simulink model "TailSitter_waypoints"  (R2018b)
settings: Solver=VariableStepAuto  StartTime=0.0  StopTime=500  RelTol=1e-3
values from neighbouring files (symbols this model uses):
  p =     [ds.mat]    (also in vxs.mat)
undefined symbols (not defined in the file or in its folder): quatnormalize
libraries: aerolibutil x18, simulink x8, sharedtransform x4, vrlib x3, sharedutil x3, simulink_extras x2, peGeneralControl x1, aerolibanim x1, aerolibanimutils x1
(part 1 of 2)
settings Model: Creator=Robert  LastModifiedBy=Robert

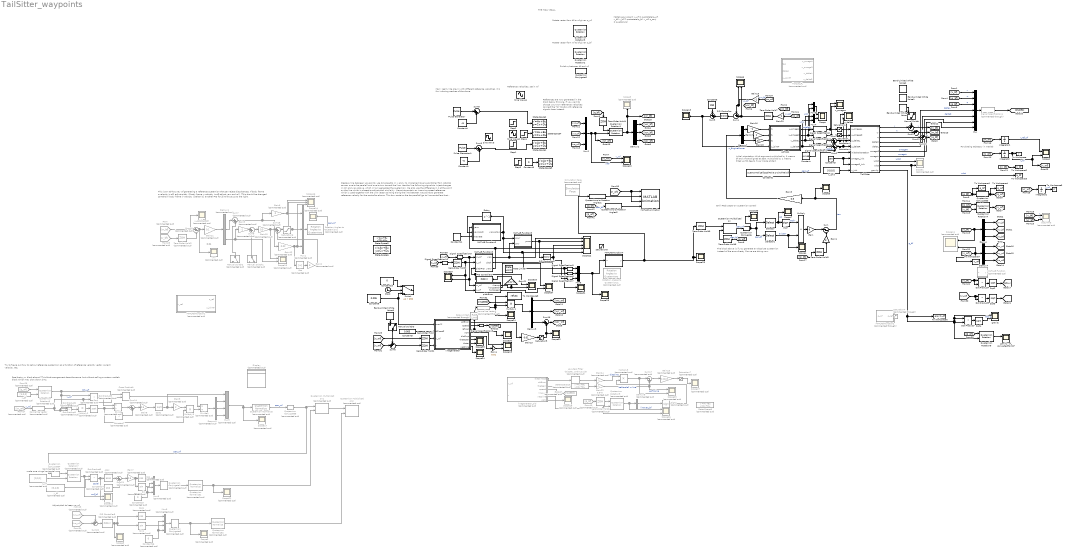
== system TailSitter_waypoints ==
  note: 0.01
  note: The block above is if you generate an absolute
      | quaternion instead of the error directy like we are doing now.
  note: References are now generated in the
      |  block below this one. If you want to
      | choose your own referrence velocities
      | connect the "to" blocks with reference
      | signals here instead.
  note: Create a line between waypoints, use 2d projectio in x and y to implement dual p-controller from robotics course, one to be paralell and one to turn toward the line.
      | Use the line following signals to inject changes in roll and yaw above, which in turn generates the quaternion.
      | We also use the difference in z at the point on the line which is closest to adjust pitch similairly.
      | Wapoints contain an incoming speed reference, which is used together with the unit vector pointing along the line between waypoints to generate reference velocity for the
      | controller above. This box contains the be parallell/go to line controllers that modify
      | the above generated signals.
      | I use low pass filters on the line vector and speed to avoid sharp jumps
      | when switching waypoints.scope
  note: Initial orientation; third argument multiplied
      | by 0 means bf and wf are aligned at start,
      | multiplied by 1 means tilted up 90 deg to
      | hiver mode at start,
  note: Man I really like playin with different reference
      | velocities, it is fun inducing crashes of the drone
  note: This is an ad-hoc way of generating a reference quaternion that can reject disturbances.
      | If body frame z-velocity is off, adjust pitch. If body frame y-velocity is off adjust yaw and roll. (This should be changed somehow)
      | body frame x-velocity is taken by another PID for joint thrust up to the right.
  note: THE HOLY GRAIL
  note: Reference velocities, set in wf
  note: For plotting trajectory in matlab
  note: Emil Fresk paper on quaternion control
  note: Rotate vector from bf to wf given q_wf
  note: Switch q between bf and wf
  note: Rotate vector from wf to bf given q_bf
  note: Matlab equivalent:
      |
      | v_wf = quatrotate(q_wf, v_bf)
      |
      |
      |
      |
      | v_bf = quatrotate(q_bf, v_wf)
      |
      |
      |
      |
      |
      |
      |
      | q_conj = quatconj(q)
  note: Adjust pitch to keep vzr_wf
  note: make sure wings horisontal
  note: See that q_uv block above? This block arangement does the same, but without calling a custom matlab block which may slow down sims.
  note: Try to figure out how to set our reference quaternion as a function of reference velocity vector, current velocity, etc.
  Abs : Abs  Commented=on
  Acos : Trigonometry  Commented=on  Operator=acos
  AdHoc1 : MATLAB Function  TreatAsAtomicUnit=on
  Band-Limited White Noise : simulink/Sources/Band-Limited White Noise  Cov=[0.01]  Ts=0.2  seed=[23343]
  Band-Limited White Noise1 : simulink/Sources/Band-Limited White Noise  Cov=[0.01]  Ts=0.1  seed=[23342]
  Band-Limited White Noise2 : simulink/Sources/Band-Limited White Noise  Cov=[0.01]  Ts=0.1  seed=[23341]
  Band-Limited White Noise3 : simulink/Sources/Band-Limited White Noise  Cov=[0.01 0.01 0.01]  Ts=p.Ts  seed=[23341]
  Clock : Clock
  Constant : Constant  Value=-0.195
  Constant1 : Constant  Value=-5
  Constant10 : Constant  Value=0  SampleTime=p.Ts
  Constant11 : Constant  Value=0.04*10
  Constant14 : Constant  Commented=on  Value=pi/2
  Constant15 : Constant  Commented=on  Value=0
  Constant16 : Constant  Commented=on  Value=0
  Constant2 : Constant  Value=quatnormalize([cosd(45),0,1*sind(45),0])  VectorParams1D=off
  Constant3 : Constant  Value=290
  Constant4 : Constant  Value=-6
  Constant5 : Constant  Value=0.005  SampleTime=p.Ts
  Constant6 : Constant  Value=290
  Constant7 : Constant  Commented=on
  Constant8 : Constant  Value=0.005  SampleTime=p.Ts
  Constant9 : Constant  Value=0
  Cos : Trigonometry  Commented=on  Operator=cos
  Cos1 : Trigonometry  Commented=on  Operator=cos
  Cross Product1 : vrlib/Utilities/Cross Product  Commented=on
      settings: SourceProductBaseCode=VR
  Delay : Delay  DelayLength=1
  Demux{,2..4,7} (5 alike) : Demux  Outputs=3
  Demux1 : Demux  Commented=on  Outputs=3
  Demux5 : Demux  Commented=on  Outputs=3
  Demux8 : Demux  Commented=on  Outputs=3
  Display : Display  Commented=on
  Divide : Product  Commented=on  Inputs=*/
  Divide1 : Product  Commented=on  Inputs=*/
  Dot Product{1..3,6} (4 alike) : DotProduct  Commented=on  InputSameDT=on  OutDataTypeStr=Inherit: Inherit via internal rule
  Dot Product4 : DotProduct  InputSameDT=on  OutDataTypeStr=Inherit: Inherit via internal rule
  Dot Product5 : DotProduct  InputSameDT=on  OutDataTypeStr=Inherit: Inherit via internal rule
  Dot Product7 : DotProduct  InputSameDT=on  OutDataTypeStr=Inherit: Inherit via internal rule
  From : From  Commented=on  GotoTag=vr_bf
  From26 : From  Commented=on  GotoTag=q_wf
  From27 : From  Commented=on  GotoTag=vr_wf
  From28 : From  Commented=on  GotoTag=v_bf
  From33 : From  Commented=on  GotoTag=vz_wf
  From34 : From  Commented=on  GotoTag=vzr_wf
  From40 : From  Commented=on  GotoTag=q_bf
  Gain : Gain  Gain=8
  Gain1 : Gain  Gain=3
  Gain11 : Gain  Commented=on  Gain=0.1
  Gain12 : Gain  Commented=on  Gain=0.02
  Gain13 : Gain  Gain=0.01
  Gain15 : Gain  Commented=on  Gain=0.5
  Gain16 : Gain  Gain=-1
  Gain17 : Gain
  Gain18 : Gain  Gain=-30
  Gain19 : Gain  Gain=-1
  Gain2 : Gain  Commented=on  Gain=5
  Gain20 : Gain  Gain=-1
  Gain21 : Gain  Gain=-0.01*0
  Gain22 : Gain  Commented=on  Gain=0.5*0
  Gain23 : Gain  Commented=on  Gain=0.0025
  Gain24 : Gain  Commented=on  Gain=-1
  Gain3 : Gain  Gain=0.5
  Gain4 : Gain  Gain=0.01
  Gain5 : Gain  Commented=on  Gain=-1
  Gain6 : Gain  Commented=on  Gain=0
  Gain7 : Gain  Commented=on  Gain=0.5
  Gain8 : Gain  Commented=on  Gain=0.5
  Gain9 : Gain  Commented=on  Gain=2
  Goto27 : Goto  Commented=on  GotoTag=rspeed
  Integrator : Integrator
  Integrator1 : Integrator
  Integrator2 : Integrator
  Low-Pass Filter (Discrete or Continuous)3 : peGeneralControl/Low-Pass Filter (Discrete or Continuous)  Commented=on  K=1  T=2  B=inf  A=-inf  Ts=-1
  MATLAB Animation : aerolibanim/MATLAB Animation  Tag=Matlab Animation 6 DOF  Vehicles=2  Geometries={'astredwedge.mat',a}  BoundingBoxCoordinates=[-50,50,-50,50,-50,50]  CameraOffset=[-150,0,-50]  CameraViewAngle=3  SampleTime=0.2  FigurePosition=[7,613,791,375]
      settings: SourceProductName=Aerospace Blockset  SourceProductBaseCode=AE
  MATLAB Function : MATLAB Function  Commented=on  TreatAsAtomicUnit=on
  MATLAB Function1 : MATLAB Function  Commented=on  TreatAsAtomicUnit=on
  MATLAB Function2 : MATLAB Function  Commented=through  TreatAsAtomicUnit=on
  MATLAB Function3 : MATLAB Function  TreatAsAtomicUnit=on
  MATLAB Function4 : MATLAB Function  TreatAsAtomicUnit=on
  MATLAB Function5 : MATLAB Function  TreatAsAtomicUnit=on
  MATLAB Function6 : MATLAB Function  TreatAsAtomicUnit=on
  Manual Switch : ManualSwitch  CurrentSetting=0
  Manual Switch1 : ManualSwitch  Commented=on  CurrentSetting=0
  Manual Switch2 : ManualSwitch  Commented=on  CurrentSetting=0
  Manual Switch3 : ManualSwitch  CurrentSetting=0
  Multiply : Product
  Multiply1 : Product
  Multiply2 : Product  Commented=on
  Multiply3 : Product  Commented=on
  Multiply5 : Product  Commented=on
  Mux : Mux  Inputs=7
  Mux1 : Mux  Commented=on  Inputs=3
  Mux2 : Mux  Inputs=3
  Mux3 : Mux  Inputs=2
  Mux4 : Mux  Inputs=2
  Mux5 : Mux  Commented=on
  Mux6 : Mux  Inputs=3
  Mux8 : Mux  Commented=on
  Mux9 : Mux  Commented=on
  Normalize Vector : vrlib/Utilities/Normalize Vector  Commented=on  maxzero=0
      settings: SourceProductName=Simulink 3D Animation  SourceProductBaseCode=VR
  Normalize Vector1 : vrlib/Utilities/Normalize Vector  Commented=through  maxzero=0
      settings: SourceProductName=Simulink 3D Animation  SourceProductBaseCode=VR
  PID Controller : simulink/Continuous/PID Controller  Controller=PID  Form=Parallel  TimeDomain=Discrete-time  SampleTime=-1  IntegratorMethod=Forward Euler  FilterMethod=Forward Euler  ControllerParametersSource=internal  P=150*2  I=50*0.5  D=50  UseFilter=off  N=100  TunerSelectOption=Transfer Function Based (PID Tuner App)  InitialConditionSource=internal  InitialConditionForIntegrator=0  InitialConditionForFilter=0  DifferentiatorICPrevScaledInput=0  ExternalReset=none  TrackingMode=off  Kt=1  LimitOutput=on  UpperSaturationLimit=4000-290  LowerSaturationLimit=-290  LinearizeAsGain=on  AntiWindupMode=clamping  Kb=1  POutMin=[]  POutMax=[]  IOutMin=[]  IOutMax=[]  DOutMin=[]  DOutMax=[]  NOutMin=[]  NOutMax=[]  SumOutMin=[]  SumOutMax=[]  SaturationOutMin=[]  SaturationOutMax=[]  PParamMin=[]  PParamMax=[]  IParamMin=[]  IParamMax=[]  DParamMin=[]  DParamMax=[]  NParamMin=[]  NParamMax=[]  KbParamMin=[]  KbParamMax=[]  KtParamMin=[]  KtParamMax=[]  KbOutMin=[]  KbOutMax=[]  KtOutMin=[]  KtOutMax=[]  IntegratorOutMin=[]  IntegratorOutMax=[]  FilterOutMin=[]  FilterOutMax=[]  SumI1OutMin=[]  SumI1OutMax=[]  SumI2OutMin=[]  SumI2OutMax=[]  SumI3OutMin=[]  SumI3OutMax=[]  SumI4OutMin=[]  SumI4OutMax=[]  SumDOutMin=[]  SumDOutMax=[]  DifferentiatorOutMin=[]  DifferentiatorOutMax=[]  FilterDiffOutCoefMin=[]  FilterDiffOutCoefMax=[]  ReciprocalOutMin=[]  ReciprocalOutMax=[]  SumDenOutMin=[]  SumDenOutMax=[]  SumNumOutMin=[]  SumNumOutMax=[]  DivideOutMin=[]  DivideOutMax=[]  IntegratorContinuousStateAttributes=''  IntegratorStateMustResolveToSignalObject=off  IntegratorRTWStateStorageClass=Auto  FilterContinuousStateAttributes=''  FilterStateMustResolveToSignalObject=off  FilterRTWStateStorageClass=Auto  ParallelPVariant=InternalParameters  IdealPVariant=Disabled  IVariant=InternalParameters  DVariant=InternalParameters  IntegratorVariant=Discrete  SatVariant=Enabled  AWVariant=DiscClampingParallel  PCopyVariant=Disabled  TRVariant=Disabled  FdbkBlocksVariant=Forward  IdealPFdbkVariant=Disabled  SatFdbkVariant=Disabled  DerivativeFilterVariant=Differentiator  NVariant=Passthrough  NCopyVariant=Disabled_SignalSpec  FilterICVariant=InternalICsDifferentiator  IntegratorICVariant=InternalICs  ExternalResetVariant=Disabled  TRSumVariant=Passthrough  SumFdbkVariant=Disabled  SumVariant=Sum_PID
  PID Controller1 : simulink/Continuous/PID Controller  Controller=PID  Form=Parallel  TimeDomain=Discrete-time  SampleTime=-1  IntegratorMethod=Forward Euler  FilterMethod=Forward Euler  ControllerParametersSource=internal  P=2*1.25*0  I=0.1*2  D=1*0  UseFilter=off  N=100  TunerSelectOption=Transfer Function Based (PID Tuner App)  InitialConditionSource=internal  InitialConditionForIntegrator=0  InitialConditionForFilter=0  DifferentiatorICPrevScaledInput=0  ExternalReset=none  TrackingMode=off  Kt=1  LimitOutput=on  UpperSaturationLimit=deg2rad(9)  LowerSaturationLimit=-deg2rad(9)  LinearizeAsGain=on  AntiWindupMode=clamping  Kb=1  POutMin=[]  POutMax=[]  IOutMin=[]  IOutMax=[]  DOutMin=[]  DOutMax=[]  NOutMin=[]  NOutMax=[]  SumOutMin=[]  SumOutMax=[]  SaturationOutMin=[]  SaturationOutMax=[]  PParamMin=[]  PParamMax=[]  IParamMin=[]  IParamMax=[]  DParamMin=[]  DParamMax=[]  NParamMin=[]  NParamMax=[]  KbParamMin=[]  KbParamMax=[]  KtParamMin=[]  KtParamMax=[]  KbOutMin=[]  KbOutMax=[]  KtOutMin=[]  KtOutMax=[]  IntegratorOutMin=[]  IntegratorOutMax=[]  FilterOutMin=[]  FilterOutMax=[]  SumI1OutMin=[]  SumI1OutMax=[]  SumI2OutMin=[]  SumI2OutMax=[]  SumI3OutMin=[]  SumI3OutMax=[]  SumI4OutMin=[]  SumI4OutMax=[]  SumDOutMin=[]  SumDOutMax=[]  DifferentiatorOutMin=[]  DifferentiatorOutMax=[]  FilterDiffOutCoefMin=[]  FilterDiffOutCoefMax=[]  ReciprocalOutMin=[]  ReciprocalOutMax=[]  SumDenOutMin=[]  SumDenOutMax=[]  SumNumOutMin=[]  SumNumOutMax=[]  DivideOutMin=[]  DivideOutMax=[]  IntegratorContinuousStateAttributes=''  IntegratorStateMustResolveToSignalObject=off  IntegratorRTWStateStorageClass=Auto  FilterContinuousStateAttributes=''  FilterStateMustResolveToSignalObject=off  FilterRTWStateStorageClass=Auto  ParallelPVariant=InternalParameters  IdealPVariant=Disabled  IVariant=InternalParameters  DVariant=InternalParameters  IntegratorVariant=Discrete  SatVariant=Enabled  AWVariant=DiscClampingParallel  PCopyVariant=Disabled  TRVariant=Disabled  FdbkBlocksVariant=Forward  IdealPFdbkVariant=Disabled  SatFdbkVariant=Disabled  DerivativeFilterVariant=Differentiator  NVariant=Passthrough  NCopyVariant=Disabled_SignalSpec  FilterICVariant=InternalICsDifferentiator  IntegratorICVariant=InternalICs  ExternalResetVariant=Disabled  TRSumVariant=Passthrough  SumFdbkVariant=Disabled  SumVariant=Sum_PID
  PID Controller2 : simulink/Continuous/PID Controller  Controller=PID  Form=Parallel  TimeDomain=Discrete-time  SampleTime=-1  IntegratorMethod=Forward Euler  FilterMethod=Forward Euler  ControllerParametersSource=internal  P=1*0  I=0  D=0.5*0  UseFilter=off  N=100  TunerSelectOption=Transfer Function Based (PID Tuner App)  InitialConditionSource=internal  InitialConditionForIntegrator=0  InitialConditionForFilter=0  DifferentiatorICPrevScaledInput=0  ExternalReset=none  TrackingMode=off  Kt=1  LimitOutput=on  UpperSaturationLimit=deg2rad(50)  LowerSaturationLimit=-deg2rad(50)  LinearizeAsGain=on  AntiWindupMode=clamping  Kb=1  POutMin=[]  POutMax=[]  IOutMin=[]  IOutMax=[]  DOutMin=[]  DOutMax=[]  NOutMin=[]  NOutMax=[]  SumOutMin=[]  SumOutMax=[]  SaturationOutMin=[]  SaturationOutMax=[]  PParamMin=[]  PParamMax=[]  IParamMin=[]  IParamMax=[]  DParamMin=[]  DParamMax=[]  NParamMin=[]  NParamMax=[]  KbParamMin=[]  KbParamMax=[]  KtParamMin=[]  KtParamMax=[]  KbOutMin=[]  KbOutMax=[]  KtOutMin=[]  KtOutMax=[]  IntegratorOutMin=[]  IntegratorOutMax=[]  FilterOutMin=[]  FilterOutMax=[]  SumI1OutMin=[]  SumI1OutMax=[]  SumI2OutMin=[]  SumI2OutMax=[]  SumI3OutMin=[]  SumI3OutMax=[]  SumI4OutMin=[]  SumI4OutMax=[]  SumDOutMin=[]  SumDOutMax=[]  DifferentiatorOutMin=[]  DifferentiatorOutMax=[]  FilterDiffOutCoefMin=[]  FilterDiffOutCoefMax=[]  ReciprocalOutMin=[]  ReciprocalOutMax=[]  SumDenOutMin=[]  SumDenOutMax=[]  SumNumOutMin=[]  SumNumOutMax=[]  DivideOutMin=[]  DivideOutMax=[]  IntegratorContinuousStateAttributes=''  IntegratorStateMustResolveToSignalObject=off  IntegratorRTWStateStorageClass=Auto  FilterContinuousStateAttributes=''  FilterStateMustResolveToSignalObject=off  FilterRTWStateStorageClass=Auto  ParallelPVariant=InternalParameters  IdealPVariant=Disabled  IVariant=InternalParameters  DVariant=InternalParameters  IntegratorVariant=Discrete  SatVariant=Enabled  AWVariant=DiscClampingParallel  PCopyVariant=Disabled  TRVariant=Disabled  FdbkBlocksVariant=Forward  IdealPFdbkVariant=Disabled  SatFdbkVariant=Disabled  DerivativeFilterVariant=Differentiator  NVariant=Passthrough  NCopyVariant=Disabled_SignalSpec  FilterICVariant=InternalICsDifferentiator  IntegratorICVariant=InternalICs  ExternalResetVariant=Disabled  TRSumVariant=Passthrough  SumFdbkVariant=Disabled  SumVariant=Sum_PID
  PID Controller5 : simulink/Continuous/PID Controller  Commented=on  Controller=PID  Form=Parallel  TimeDomain=Continuous-time  SampleTime=-1  IntegratorMethod=Forward Euler  FilterMethod=Forward Euler  ControllerParametersSource=internal  P=0.04*2  I=0  D=0  UseFilter=on  N=100  TunerSelectOption=Transfer Function Based (PID Tuner App)  InitialConditionSource=internal  InitialConditionForIntegrator=0  InitialConditionForFilter=0  DifferentiatorICPrevScaledInput=0  ExternalReset=none  TrackingMode=off  Kt=1  LimitOutput=off  UpperSaturationLimit=inf  LowerSaturationLimit=-inf  LinearizeAsGain=on  AntiWindupMode=none  Kb=1  POutMin=[]  POutMax=[]  IOutMin=[]  IOutMax=[]  DOutMin=[]  DOutMax=[]  NOutMin=[]  NOutMax=[]  SumOutMin=[]  SumOutMax=[]  SaturationOutMin=[]  SaturationOutMax=[]  PParamMin=[]  PParamMax=[]  IParamMin=[]  IParamMax=[]  DParamMin=[]  DParamMax=[]  NParamMin=[]  NParamMax=[]  KbParamMin=[]  KbParamMax=[]  KtParamMin=[]  KtParamMax=[]  KbOutMin=[]  KbOutMax=[]  KtOutMin=[]  KtOutMax=[]  IntegratorOutMin=[]  IntegratorOutMax=[]  FilterOutMin=[]  FilterOutMax=[]  SumI1OutMin=[]  SumI1OutMax=[]  SumI2OutMin=[]  SumI2OutMax=[]  SumI3OutMin=[]  SumI3OutMax=[]  SumI4OutMin=[]  SumI4OutMax=[]  SumDOutMin=[]  SumDOutMax=[]  DifferentiatorOutMin=[]  DifferentiatorOutMax=[]  FilterDiffOutCoefMin=[]  FilterDiffOutCoefMax=[]  ReciprocalOutMin=[]  ReciprocalOutMax=[]  SumDenOutMin=[]  SumDenOutMax=[]  SumNumOutMin=[]  SumNumOutMax=[]  DivideOutMin=[]  DivideOutMax=[]  IntegratorContinuousStateAttributes=''  IntegratorStateMustResolveToSignalObject=off  IntegratorRTWStateStorageClass=Auto  FilterContinuousStateAttributes=''  FilterStateMustResolveToSignalObject=off  FilterRTWStateStorageClass=Auto  ParallelPVariant=InternalParameters  IdealPVariant=Disabled  IVariant=InternalParameters  DVariant=InternalParameters  IntegratorVariant=Continuous  SatVariant=Disabled  AWVariant=Passthrough  PCopyVariant=Disabled  TRVariant=Disabled  FdbkBlocksVariant=Forward  IdealPFdbkVariant=Disabled  SatFdbkVariant=Disabled  DerivativeFilterVariant=ContFilter  NVariant=InternalParameters  NCopyVariant=Disabled  FilterICVariant=InternalICsFilter  IntegratorICVariant=InternalICs  ExternalResetVariant=Disabled  TRSumVariant=Passthrough  SumFdbkVariant=Disabled  SumVariant=Sum_PID
  Pulse Generator : DiscretePulseGenerator  PulseType=Time based  Amplitude=12  Period=50  PulseWidth=50
  Pulse Generator1 : DiscretePulseGenerator  PulseType=Time based  Amplitude=8  Period=60  PulseWidth=50  PhaseDelay=30
  Quaternion Conjugate : aerolibutil/Quaternion Conjugate
      settings: SourceProductName=Aerospace Blockset  SourceProductBaseCode=AE
  Quaternion Conjugate{1,4..6} (4 alike) : aerolibutil/Quaternion Conjugate  Commented=on
      settings: SourceProductName=Aerospace Blockset  SourceProductBaseCode=AE
  Quaternion Conjugate2 : aerolibutil/Quaternion Conjugate
      settings: SourceProductName=Aerospace Blockset  SourceProductBaseCode=AE
  Quaternion Conjugate3 : aerolibutil/Quaternion Conjugate
      settings: SourceProductName=Aerospace Blockset  SourceProductBaseCode=AE
  Quaternion Multiplication : aerolibutil/Quaternion Multiplication
  Quaternion Multiplication1 : aerolibutil/Quaternion Multiplication  Commented=on
  Quaternion Multiplication2 : aerolibutil/Quaternion Multiplication  Commented=on
  Quaternion Normalize : sharedutil/Quaternion Normalize  Commented=on  aMode=aMode
      settings: SourceProductName=Aerospace Blockset  SourceProductBaseCode=AE
  Quaternion Normalize1 : sharedutil/Quaternion Normalize  Commented=on  aMode=aMode
      settings: SourceProductName=Aerospace Blockset  SourceProductBaseCode=AE
  Quaternion Normalize2 : sharedutil/Quaternion Normalize  Commented=on  aMode=aMode
      settings: SourceProductName=Aerospace Blockset  SourceProductBaseCode=AE
  Quaternion Rotation{1..4,8} (5 alike) : aerolibutil/Quaternion Rotation
  Quaternion Rotation5 : aerolibutil/Quaternion Rotation  Commented=on
  Quaternion Rotation7 : aerolibutil/Quaternion Rotation  Commented=on
  Quaternion Rotation9 : aerolibutil/Quaternion Rotation  Commented=on
  Quaternions to Rotation Angles1 : sharedtransform/Quaternions to Rotation Angles  rotationOrder=XYZ  aMode=aMode
      settings: SourceProductBaseCode=AE
  Quaternions to Rotation Angles2 : sharedtransform/Quaternions to Rotation Angles  rotationOrder=XYZ  aMode=aMode
      settings: SourceProductBaseCode=AE
  Rate Limiter : RateLimiter  RisingSlewLimit=0.1  FallingSlewLimit=-0.1  SampleTimeMode=inherited
  Rate Limiter1 : RateLimiter  Commented=through  RisingSlewLimit=0.03  FallingSlewLimit=-0.03  SampleTimeMode=inherited
  Rotation Angles to Quaternions : sharedtransform/Rotation Angles to Quaternions  Commented=on  rotationOrder=ZYX  aMode=aMode
      settings: SourceProductName=Aerospace Blockset  SourceProductBaseCode=AE
  Rotation Angles to Quaternions1 : sharedtransform/Rotation Angles to Quaternions  Commented=on  rotationOrder=ZYX  aMode=aMode
      settings: SourceProductName=Aerospace Blockset  SourceProductBaseCode=AE
  Saturation : Saturate  UpperLimit=1000  LowerLimit=0
  Saturation1 : Saturate  UpperLimit=1000  LowerLimit=0
  Saturation2 : Saturate  UpperLimit=1  LowerLimit=-1
  Saturation3 : Saturate  UpperLimit=1  LowerLimit=-1
  Saturation4 : Saturate  Commented=through
  Saturation5 : Saturate  UpperLimit=0.01  LowerLimit=-0.01
  Saturation6 : Saturate  Commented=on  UpperLimit=1  LowerLimit=-1
  Saturation7 : Saturate  Commented=on
  Saturation8 : Saturate  UpperLimit=deg2rad(50)  LowerLimit=-deg2rad(50)
  Scope{,2,6,10,19..20,29,33,37} (9 alike) : Scope  NumInputPorts=2
  Scope{1,11..12,15,23,26} (6 alike) : Scope  Commented=on  NumInputPorts=2
  Scope{4..5,7,13,24..25,28,30..32,34..35} (12 alike) : Scope
  Scope{3,8..9,14,17..18,21,27} (8 alike) : Scope  Commented=on
  Scope16 : Scope  Commented=on  NumInputPorts=3
  Scope22 : Scope  NumInputPorts=5
  Selector : Selector  IndexMode=Zero-based  InputPortWidth=4  IndexOptions=Index vector (dialog)  Indices=[0 ]  OutputSizes=1
  Selector1 : Selector  IndexMode=Zero-based  InputPortWidth=4  IndexOptions=Index vector (dialog)  Indices=[1:3]  OutputSizes=1
  Sign : Signum
  Sign2 : Signum  Commented=on
  Signal Specification{,1..3,5..8} (8 alike) : SignalSpecification  Dimensions=1
  Signal Specification10 : SignalSpecification  Dimensions=3
  Signal Specification4 : SignalSpecification  Commented=through  Dimensions=14
  Signal Specification9 : SignalSpecification  Dimensions=3
  Simulation Pace : aerolibanimutils/Simulation Pace  Commented=on  SimulationPace=2  SleepMode=Auto  OutputPaceError=off  SampleTime=1/30
  Sin : Trigonometry  Commented=on
  Sin1 : Trigonometry  Commented=on
  Sine Wave : Sin  Amplitude=-2  Frequency=1/15  Phase=pi/2  SampleTime=0
  Sine Wave1 : Sin  Amplitude=-8  Frequency=1/20  SampleTime=0
  Sine Wave2 : Sin  Amplitude=10  Frequency=1/45  SampleTime=0
  Sqrt : Sqrt  Commented=on  SaturateOnIntegerOverflow=on
  Sqrt1 : Sqrt  Commented=on  SaturateOnIntegerOverflow=on
  Sqrt2 : Sqrt  SaturateOnIntegerOverflow=on
  Sqrt3 : Sqrt  SaturateOnIntegerOverflow=on
  Sqrt4 : Sqrt  SaturateOnIntegerOverflow=on
  State-Space1 : StateSpace  A=-1/5  B=1/5  D=0  InitialCondition=0
  State-Space10 : StateSpace  Commented=on  A=-1/15  B=1/15  D=0  InitialCondition=0
  State-Space2 : StateSpace  A=-1/15  B=1/15  D=0  InitialCondition=0
  State-Space3 : StateSpace  A=-1/15  B=1/15  D=0  InitialCondition=0
  State-Space4 : StateSpace  A=-1/15  B=1/15  D=0  InitialCondition=0
  State-Space5 : StateSpace  A=-1/5  B=1/5  D=0  InitialCondition=0
  State-Space6 : StateSpace  A=-1/2*eye(3)  B=1/2*eye(3)  C=eye(3)  D=0*eye(3)  InitialCondition=0
  State-Space9 : StateSpace  Commented=on  A=-1/4  B=1/4  D=0  InitialCondition=0
  Step1 : Step  Time=20  After=-10  SampleTime=0
  Step2 : Step  Time=100  After=5  SampleTime=0
  Step3 : Step  Time=30  Before=-1  After=0  SampleTime=0
  Step4 : Step  Time=60  After=18  SampleTime=0
  Sum : Sum  Inputs=|--
  Sum{1..3,8,16} (5 alike) : Sum  Inputs=|++
  Sum10 : Sum  Commented=on  Inputs=|+-
  Sum{5..6,11..13} (5 alike) : Sum  Inputs=++|
  Sum{7,9,14..15} (4 alike) : Sum  Commented=on  Inputs=|++
  Sum17 : Sum  Commented=on  Inputs=|-+
  Sum21 : Sum  Commented=on  Inputs=|+-
  Sum22 : Sum  Commented=on  Inputs=-+|
  Sum4 : Sum  Inputs=+-|
  Switch : Switch  Criteria=u2 > Threshold  Threshold=250
  TailSitter : Subsystem
  To Workspace : ToWorkspace  VariableName=r  SaveFormat=Timeseries  SampleTime=p.Ts_log
  To Workspace1 : ToWorkspace  VariableName=q_bf  SaveFormat=Timeseries  SampleTime=p.Ts_log
  To Workspace2 : ToWorkspace  VariableName=v_bf  SaveFormat=Timeseries  SampleTime=p.Ts_log
  To Workspace3 : ToWorkspace  VariableName=a_bf  SaveFormat=Timeseries  SampleTime=p.Ts_log
  To Workspace4 : ToWorkspace  VariableName=q_wf  SaveFormat=Timeseries  SampleTime=p.Ts_log
  To Workspace5 : ToWorkspace  VariableName=rr  SaveFormat=Timeseries  SampleTime=p.Ts_log
  To Workspace6 : ToWorkspace  VariableName=gravity_bf  SaveFormat=Timeseries  SampleTime=p.Ts_log
  To Workspace7 : ToWorkspace  VariableName=v_wf  SaveFormat=Timeseries  SampleTime=p.Ts_log
  To Workspace8 : ToWorkspace  VariableName=refvec  SaveFormat=Timeseries  SampleTime=p.Ts_log
  Torque_FL : MATLAB Function  Commented=on  TreatAsAtomicUnit=on
  Zero-Order Hold{,1,3..5,7..9} (8 alike) : ZeroOrderHold  SampleTime=p.Ts
  Zero-Order Hold2 : ZeroOrderHold  Commented=on  SampleTime=p.Ts
  Zero-Order Hold6 : ZeroOrderHold  Commented=on  SampleTime=p.Ts
  bodyfrme : Scope  Commented=on  NumInputPorts=2
  gravity : Scope  NumInputPorts=2
  gravity_wf_convertedfrombf : Scope  NumInputPorts=2
  linegenerator : MATLAB Function  TreatAsAtomicUnit=on
  linegenerator_old : MATLAB Function  Commented=on  TreatAsAtomicUnit=on
  pitchError : MATLAB Function  TreatAsAtomicUnit=on
  u_deltas : Scope  NumInputPorts=2
  u_omegas : Scope  NumInputPorts=2
  v_isnit : Constant  Value=[0,0,0]
  "v_ref_bf_attctrl " : Scope  Commented=on
  vr-v : Scope  Commented=on
  x_bf : Constant  Commented=on  Value=[1,0,0]
  y_bf : Constant  Commented=on  Value=[0,1,0]
  z_wf : Constant  Commented=on  Value=[0,0,1]
  wires:
  Selector1/1 -> Scope4/1, Multiply/2  "axiserr"
  Selector/1 -> Scope7/1, Sign/1  "q0"
  Sign/1 -> Multiply/1  "rotdir"
  Gain1/1 -> Sum/2
  Sum5/1 -> AdHoc1/4(u_jointT), Scope13/1  "u_EnginePower"
  Constant3/1 -> TailSitter/7(omegaR_init), TailSitter/6(omegaL_init)
  Sum11/1 -> [v_bf]  "v"
  TailSitter/8(wdot) -> Scope1/1  "wdot"
  TailSitter/9(vdot) -> To Workspace3/1, Scope1/2  "vdot"
  Integrator/1 -> [r_wf], Scope2/2, To Workspace/1  "r_wf"
  [v_wf] -> Integrator/1
  v_isnit/1 -> TailSitter/8(v_init)
  Sum4/1 -> PID Controller/1
  Sum/1 -> Scope5/1, Gain3/1  "tao"
  PID Controller/1 -> Sum5/2
  Constant6/1 -> Sum5/1
  Multiply/1 -> Gain/1
  [vzr_wf] -> Gain19/1  "vxr_bf"
  Saturation/1 -> TailSitter/2(u_omegaR)
  Saturation1/1 -> TailSitter/1(u_omegaL)
  TailSitter/3(q) -> Sum13/2
  Mux2/1 -> Scope10/2, [vr_wf], Quaternion Rotation1/2  "vref"
  Quaternion Rotation1/1 -> Demux2/1, [vr_bf], Scope9/1
  Demux2/3 -> [vzr_bf]
  Demux2/2 -> [vyr_bf]
  Demux2/1 -> [vxr_bf]
  Zero-Order Hold7/1 -> Scope6/2, Sum4/2  "vx_bf"
  [v_wf] -> Scope10/1  "v_wf"
  [q_bf] -> Zero-Order Hold4/1
  [q_bf] -> To Workspace1/1, Quaternion Conjugate3/1
  Quaternion Conjugate3/1 -> To Workspace4/1, [q_wf]
  [vxr_wf] -> Mux2/1
  [vyr_wf] -> Mux2/2
  [vzr_wf] -> Mux2/3
  [q_wf] -> Quaternion Rotation4/1
  Quaternion Rotation4/1 -> [v_wf]
  [v_bf] -> Quaternion Rotation4/2
  TailSitter/2(w) -> Sum12/2  "w"
  Demux/1 -> [vx_bf]
  Demux/3 -> [vz_bf]
  Demux/2 -> [vy_bf]
  [v_bf] -> Scope11/1, Demux/1
  Demux4/2 -> [vy_wf]
  Demux4/3 -> [vz_wf]
  Demux4/1 -> [vx_wf]
  [v_wf] -> To Workspace7/1, Scope11/2, Demux4/1
  [v_bf] -> To Workspace2/1
  [v_bf] -> Dot Product4/2, Dot Product4/1
  Sqrt2/1 -> [abs_v]
  [vr_wf] -> Integrator1/1
  Integrator1/1 -> Scope2/1  "r_ref_wf"
  [w_bf] -> Zero-Order Hold5/1
  [v_bf] -> bodyfrme/1  "v"
  [vr_bf] -> bodyfrme/2  "vr"
  [vr_wf] -> Integrator2/1
  Integrator2/1 -> To Workspace5/1  "r_wf"
  Dot Product4/1 -> Sqrt2/1
  Gain/1 -> Sum/1
  Constant2/1 -> TailSitter/5(initialOrientation)  "qerr_wf"
  [v_bf] -> Mux/1  "v"
  [w_bf] -> Mux/2  "w"
  [q_bf] -> Mux/3  "q"
  TailSitter/5(deltaL) -> Mux/4  "deltaL"
  TailSitter/4(deltaR) -> Mux/5  "deltaR"
  TailSitter/7(omegaL) -> Mux/6  "omegaL"
  TailSitter/6(omegaR) -> Mux/7  "omegaR"
  AdHoc1/1(u_omegaL) -> Mux3/2, Signal Specification/1  "uWL"
  AdHoc1/2(u_omegaR) -> Mux3/1, Signal Specification1/1
  AdHoc1/3(u_deltaL) -> Mux4/1, Signal Specification2/1  "uWL"
  AdHoc1/4(u_deltaR) -> Signal Specification3/1, Mux4/2  "udeltaL"
  Signal Specification/1 -> u_omegas/1, Saturation1/1
  Signal Specification1/1 -> u_omegas/2, Saturation/1
  Signal Specification2/1 -> Sum1/1
  Signal Specification3/1 -> Sum2/1
  Mux/1 -> Signal Specification4/1
  Sum1/1 -> Saturation2/1
  Signal Specification4/1 -> [states]
  Acos/1 -> Sum21/1
  y_bf/1 -> Dot Product6/2
  Multiply3/1 -> Divide1/2
  Sum22/1 -> PID Controller5/1
  Dot Product3/1 -> Divide/1
  Demux5/2 -> Mux5/3
  Quaternion Conjugate6/1 -> Scope3/1, Quaternion Normalize2/1
  Mux5/1 -> Scope17/1, Quaternion Normalize/1
  From33/1 -> Sum22/1
  Constant15/1 -> Mux8/3, Mux8/4
  Mux8/1 -> Quaternion Conjugate1/1
  Demux5/1 -> Mux5/2
  PID Controller5/1 -> Scope8/1, Cos1/1, Sin1/1
  From27/1 -> Normalize Vector/1  "v_wf"
  Cos1/1 -> Mux9/1
  Quaternion Rotation7/1 -> Scope12/1, Dot Product6/1  "zwf_bf"
  Constant16/1 -> Mux9/2, Mux9/4
  Quaternion Normalize1/1 -> Scope21/1, Quaternion Multiplication1/2
  Gain7/1 -> Sin/1, Cos/1
  Sum21/1 -> Gain7/1
  From34/1 -> Sum22/2
  Mux9/1 -> Quaternion Conjugate6/1
  Cos/1 -> Mux8/1
  Constant14/1 -> Sum21/2
  Sin/1 -> Mux8/2
  Quaternion Normalize2/1 -> Quaternion Multiplication2/2
  Multiply2/1 -> Sqrt/1
  Divide/1 -> Sum14/1
  Quaternion Conjugate1/1 -> Quaternion Normalize1/1
  Sin1/1 -> Mux9/3
  Sqrt1/1 -> Mux5/1, Gain9/1
  Quaternion Conjugate4/1 -> Quaternion Rotation7/1
  Normalize Vector/1 -> Cross Product1/2, Dot Product3/2, Dot Product2/1, Dot Product2/2  "v_wf"
  Quaternion Normalize/1 -> Quaternion Conjugate5/1  "qerr_wf"
  Gain8/1 -> Sqrt1/1
  Cross Product1/1 -> Divide1/1
  Divide1/1 -> Demux5/1
  From26/1 -> Quaternion Rotation5/1
  Sum14/1 -> Gain8/1
  z_wf/1 -> Quaternion Rotation7/2
  Dot Product6/1 -> Scope12/2, Acos/1  "cos(a)"
  Gain9/1 -> Multiply3/1
  Dot Product1/1 -> Multiply2/1
  Constant7/1 -> Sum14/2
  Dot Product2/1 -> Multiply2/2
  Sqrt/1 -> Multiply3/2, Divide/2
  Quaternion Rotation5/1 -> Dot Product3/1, Dot Product1/2, Dot Product1/1, Cross Product1/1  "bfx_wf"
  Demux5/3 -> Mux5/4
  x_bf/1 -> Quaternion Rotation5/2
  Quaternion Multiplication1/1 -> Quaternion Multiplication2/1
  Quaternion Conjugate5/1 -> Quaternion Conjugate4/1, Quaternion Multiplication1/1  "qerr_wf"
  Mux1/1 -> Rotation Angles to Quaternions/1
  From28/1 -> Zero-Order Hold2/1
  Sum10/1 -> vr-v/1, Gain11/1
  Demux1/3 -> Gain5/1, Scope15/2
  Gain5/1 -> Sum9/1
  Sum7/1 -> Gain12/1, Gain6/1
  Gain6/1 -> Scope16/1, Mux1/1
  Gain15/1 -> Sum15/1, Scope15/1
  Gain11/1 -> Demux1/1
  Saturation2/1 -> u_deltas/1, TailSitter/3(u_deltaL)
  Sum2/1 -> Saturation3/1
  Saturation3/1 -> u_deltas/2, TailSitter/4(u_deltaR)
  Constant/1 -> Sum2/2, Sum1/2  "udeltaL"
  Sum3/1 -> State-Space1/1
  Gain12/1 -> Abs/1, Scope16/3, Mux1/3
  Dot Product5/1 -> Sqrt3/1
  Sqrt3/1 -> [abs_vr]
  [vr_wf] -> Dot Product5/2, Dot Product5/1
  From/1 -> "v_ref_bf_attctrl "/1, Sum10/1
  Sum8/1 -> State-Space2/1
  Step4/1 -> State-Space4/1
  TailSitter/10(gravity) -> To Workspace6/1, gravity/1, Dot Product7/1, Quaternion Rotation8/2, Dot Product7/2  "g_bf"
  Dot Product7/1 -> Sqrt4/1
  [q_wf] -> Quaternion Rotation8/1
  Quaternion Rotation8/1 -> gravity_wf_convertedfrombf/1
  Pulse Generator1/1 -> Sum3/1
  Constant1/1 -> Sum3/2
  Pulse Generator/1 -> Sum8/1
  Constant4/1 -> Sum8/2
  Sqrt4/1 -> gravity/2  "abs g"
  Gain3/1 -> Demux7/1
  [v_wf] -> Zero-Order Hold/1
  [r_wf] -> Sum6/2
  linegenerator/2(rspeed) -> Signal Specification8/1
  Demux3/1 -> [vxr_wf]
  Multiply1/1 -> Demux3/1
  Demux1/2 -> Sum7/1
  linegenerator/1(altError) -> Gain13/1
  Gain13/1 -> Saturation5/1
  linegenerator/4(wpN) -> Scope19/1
  Demux3/3 -> Sum16/1
  ? -> Saturation4/1
  Sum9/1 -> Gain15/1
  linegenerator/3(refvec) -> Scope30/1, Rate Limiter1/1
  [rspeed] -> Multiply1/1
  Saturation6/1 -> Scope16/2, Mux1/2
  Constant9/1 -> State-Space3/1
  TailSitter/1(v) -> Sum11/2  "v"
  Sum12/1 -> [w_bf]  "v"
  Sum13/1 -> [q_bf]  "v"
  Band-Limited White Noise/1 -> Manual Switch/1
  Manual Switch/1 -> Sum11/1
  Zero-Order Hold/1 -> linegenerator/3(v_wf)
  Zero-Order Hold1/1 -> linegenerator/4(r)
  Zero-Order Hold2/1 -> Sum10/2
  Zero-Order Hold4/1 -> Quaternion Rotation1/1
  Zero-Order Hold5/1 -> Gain1/1
  [vz_wf] -> Gain20/1  "vx_bf"
  Manual Switch1/1 -> Sum9/2
  Manual Switch2/1 -> Sum7/2
  Zero-Order Hold9/1 -> Quaternion Multiplication/1
  Rotation Angles to Quaternions/1 -> Scope14/1  "qerr_wf"
  Demux7/1 -> Gain16/1
  Demux7/2 -> Gain17/1
  Demux7/3 -> Gain18/1
  Gain16/1 -> AdHoc1/1(tx)
  Gain17/1 -> AdHoc1/2(ty)
  Gain18/1 -> AdHoc1/3(tz)
  Mux4/1 -> Scope/2
  Mux3/1 -> Scope/1
  Abs/1 -> Gain2/1
  Sum15/1 -> Saturation6/1
  Gain2/1 -> Sum15/2
  Quaternion Multiplication/1 -> Quaternion Conjugate/1  "qerr_wf"
  Gain19/1 -> Sum4/1, Scope6/1
  Gain20/1 -> Zero-Order Hold7/1
  Mux6/1 -> MATLAB Function4/1(u), Scope28/1
  [vr_wf] -> Signal Specification9/1
  Zero-Order Hold3/1 -> Scope29/1, pitchError/2(v_wf), MATLAB Function3/2(v_wf)
  pitchError/1(vherror) -> Scope20/2, Gain21/1
  Gain21/1 -> PID Controller1/1
  MATLAB Function3/2(pitch) -> Signal Specification6/1
  Sum16/1 -> [vzr_wf]
  Gain22/1 -> Scope23/1, Sum17/2  "beParalell w line"
  Low-Pass Filter (Discrete or Continuous)3/1 -> Gain24/1
  linegenerator_old/1(dist2line2d) -> Low-Pass Filter (Discrete or Continuous)3/1
  linegenerator_old/4(rspeed) -> Goto27/1
  Demux8/2 -> Sign2/1
  linegenerator_old/6(vec2line) -> Quaternion Rotation9/2, Scope26/2
  From40/1 -> Zero-Order Hold6/1
  Saturation7/1 -> Scope27/1
  State-Space10/1 -> Gain22/1
  Gain24/1 -> Multiply5/1  "dist2line"
  Quaternion Rotation9/1 -> Scope26/1, Demux8/1  "linevec_bf"
  Sign2/1 -> Multiply5/2
  linegenerator_old/7(wpN) -> Scope18/1
  Zero-Order Hold6/1 -> Quaternion Rotation9/1
  Multiply5/1 -> Scope23/2, Sum17/1  "goToLine"
  Gain23/1 -> Saturation7/1
  Sum17/1 -> Gain23/1
  linegenerator_old/3(thetaerr) -> State-Space10/1
  Constant5/1 -> linegenerator/2(d2lcoeff)
  PID Controller1/1 -> Scope20/1, MATLAB Function3/3(pitchPID)
  linegenerator/5(dist2wp) -> Gain4/1
  PID Controller2/1 -> Signal Specification7/1, Scope22/3
  MATLAB Function6/1(yawr_slow) -> MATLAB Function5/1(yawr), Scope22/5, Scope31/1, Signal Specification5/1, Delay/1
  MATLAB Function5/1(yawe) -> PID Controller2/1, Scope22/2
  MATLAB Function3/1(yaw) -> MATLAB Function5/2(yaw), Scope22/1
  Signal Specification5/1 -> Mux6/1
  Signal Specification6/1 -> Mux6/2
  Signal Specification7/1 -> Mux6/3
  Signal Specification8/1 -> [rspeed]
  Signal Specification9/1 -> Scope29/2, pitchError/1(vr_wf), MATLAB Function3/1(vr_wf)
  Signal Specification10/1 -> Zero-Order Hold3/1
  Demux3/2 -> [vyr_wf]
  Band-Limited White Noise3/1 -> Manual Switch3/1
  Sum6/1 -> Zero-Order Hold1/1
  Manual Switch3/1 -> Sum6/1
  [v_wf] -> Signal Specification10/1
  linegenerator/6(thetastar) -> Scope33/1
  linegenerator/7(theta) -> Scope33/2
  linegenerator/8(vec2line) -> Scope34/1
  Rate Limiter1/1 -> Normalize Vector1/1
  Clock/1 -> Switch/2
  Constant10/1 -> Switch/1
  Delay/1 -> MATLAB Function6/2(yawr_last)
  Constant11/1 -> MATLAB Function6/3(maxrate)
  MATLAB Function3/3(yawr) -> MATLAB Function6/1(yawr), Scope22/4
  Constant8/1 -> Switch/3, linegenerator/1(max2l)
  Saturation5/1 -> Scope32/1, Sum16/2
  Normalize Vector1/1 -> To Workspace8/1, Multiply1/2, Scope24/1
  ? -> ?
  Quaternion Conjugate/1 -> Scope35/1, Selector1/1, Selector/1  "qerr_bf"
  pitchError/2(horzspeedr) -> Scope37/1
  pitchError/3(horzspeed) -> Scope37/2
  Quaternions to Rotation Angles1/1 -> MATLAB Animation/2
  [r_wf] -> MATLAB Animation/3, MATLAB Animation/1
  Quaternions to Rotation Angles2/1 -> MATLAB Animation/4
  Zero-Order Hold8/1 -> Quaternion Multiplication/2
  Gain4/1 -> Scope19/2
  MATLAB Function4/1(y) -> Quaternions to Rotation Angles1/1, Zero-Order Hold9/1, Scope25/1
  [q_wf] -> Zero-Order Hold8/1  "qerr_bf"
  [q_bf] -> Quaternions to Rotation Angles2/1  "qerr_bf"

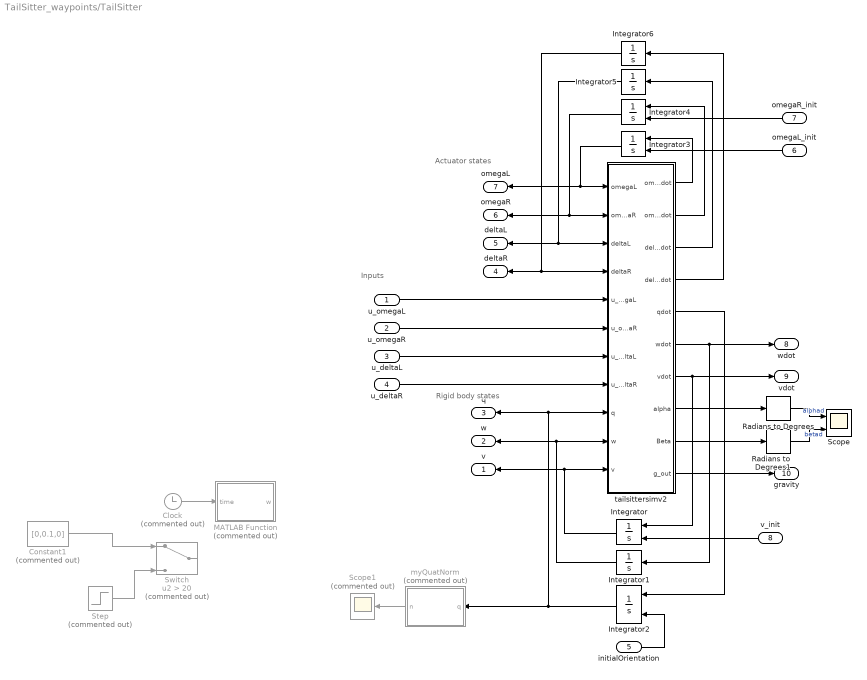
== system TailSitter_waypoints/TailSitter ==
  note: Actuator
      | states
  note: Rigid
      | body
      | states
  note: Inputs
  u_omegaL : Inport
  u_omegaR : Inport  Port=2
  u_deltaL : Inport  Port=3
  u_deltaR : Inport  Port=4
  initialOrientation : Inport  Port=5
  omegaL_init : Inport  Port=6
  omegaR_init : Inport  Port=7
  v_init : Inport  Port=8
  Clock : Clock  Commented=on
  Constant1 : Constant  Commented=on  Value=[0,0.1,0]
  Integrator : Integrator  InitialConditionSource=external  InitialCondition=[0,0,0]
  Integrator1 : Integrator  InitialCondition=[0,0,0]
  Integrator2 : Integrator  InitialConditionSource=external
  Integrator3 : Integrator  InitialConditionSource=external
  Integrator4 : Integrator  InitialConditionSource=external
  Integrator5 : Integrator
  Integrator6 : Integrator
  MATLAB Function : MATLAB Function  Commented=on  TreatAsAtomicUnit=on
  Radians to Degrees : simulink_extras/Transformations/Radians to Degrees
  Radians to Degrees1 : simulink_extras/Transformations/Radians to Degrees
  Scope : Scope  NumInputPorts=2
  Scope1 : Scope  Commented=on
  Step : Step  Commented=on  Time=10  Before=[0.1,0,0]  After=[0,0,0.1]  SampleTime=0
  Switch : Switch  Commented=on  Criteria=u2 > Threshold  Threshold=20
  myQuatNorm : MATLAB Function  Commented=on  TreatAsAtomicUnit=on
  tailsittersimv2 : MATLAB Function  TreatAsAtomicUnit=on
  v : Outport
  w : Outport  Port=2
  q : Outport  Port=3
  deltaR : Outport  Port=4
  deltaL : Outport  Port=5
  omegaR : Outport  Port=6
  omegaL : Outport  Port=7
  wdot : Outport  Port=8  PortDimensions=3
  vdot : Outport  Port=9  PortDimensions=3
  gravity : Outport  Port=10  PortDimensions=3
  wires:
  tailsittersimv2/7(vdot) -> Integrator/1, vdot/1
  tailsittersimv2/6(wdot) -> Integrator1/1, wdot/1
  tailsittersimv2/5(qdot) -> Integrator2/1
  Integrator2/1 -> tailsittersimv2/9(q), q/1, myQuatNorm/1(q)
  initialOrientation/1 -> Integrator2/2
  tailsittersimv2/1(omegaLdot) -> Integrator3/1
  Integrator3/1 -> tailsittersimv2/1(omegaL), omegaL/1
  tailsittersimv2/2(omegaRdot) -> Integrator4/1
  tailsittersimv2/3(deltaLdot) -> Integrator5/1
  tailsittersimv2/4(deltaRdot) -> Integrator6/1
  Integrator5/1 -> tailsittersimv2/3(deltaL), deltaL/1
  Integrator6/1 -> tailsittersimv2/4(deltaR), deltaR/1
  Integrator4/1 -> tailsittersimv2/2(omegaR), omegaR/1
  omegaL_init/1 -> Integrator3/2
  omegaR_init/1 -> Integrator4/2
  u_omegaL/1 -> tailsittersimv2/5(u_omegaL)
  u_omegaR/1 -> tailsittersimv2/6(u_omegaR)
  u_deltaL/1 -> tailsittersimv2/7(u_deltaL)
  u_deltaR/1 -> tailsittersimv2/8(u_deltaR)
  tailsittersimv2/8(alpha) -> Radians to Degrees/1
  Radians to Degrees/1 -> Scope/1  "alphad"
  myQuatNorm/1(n) -> Scope1/1
  Integrator/1 -> tailsittersimv2/11(v), v/1
  Clock/1 -> MATLAB Function/1(time)
  Constant1/1 -> Switch/1
  Step/1 -> Switch/3
  Integrator1/1 -> tailsittersimv2/10(w), w/1
  v_init/1 -> Integrator/2
  tailsittersimv2/9(Beta) -> Radians to Degrees1/1
  Radians to Degrees1/1 -> Scope/2  "betad"
  tailsittersimv2/10(g_out) -> gravity/1

== matlab function TailSitter_waypoints/Torque_FL ==
  data: u_omegaL output; u_omegaR output; u_deltaL output; u_deltaR output; tao input; states input; u_jointT input; p parameter
function [u_omegaL,u_omegaR, u_deltaL,u_deltaR]  = FL_torques(tao, states, u_jointT, p)


wxr = tao(1); % I wonder if this comversion from omega to tao is right? Depends on Emil Fresk implementation
wyr = tao(2);
wzr = tao(3);
v = states(1:3);
vx = v(1);
vy = v(2);
vz = v(3);
w = states(4:6);
wx = w(1);
wy = w(2);
wz = w(3);
q = states(7:10); % Possibly not needed?
q0=q(1);
q1=q(2);
q2=q(3);
q3=(4);
deltaL = states(11);
deltaR = states(12);
omegaL = states(13);
omegaR = states(14);

% init output vector
u_deltaL = 0;
u_deltaR = 0;
u_omegaL = 0;
u_omegaR = 0;

% If you know of a better way (not counting modifying the code below to use
% p.x notation, plese feel welcome to tell me.
%P = struct2cell(p);
%Pn = fieldnames(p);
%for i=1:numel(P)
%    eval(Pn{i}+"="+string(P{i})+";")
%end
Ts=p.Ts;
m=p.m;
Ix=p.Ix;
Iy=p.Iy;
Iz=p.Iz;
I=p.I;
g=p.g;
rho=p.rho;
propd=p.propd;
K_T=p.K_T;
K_v=p.K_v;
b_w=p.b_w;
Sa=p.Sa;
Saw=p.Saw;
CLdelta=p.CLdelta;
CDdelta=p.CDdelta;
SW=p.SW;
Sw_w=p.Sw_w;
Sw=p.Sw;
b=p.b;
Cmyl=p.Cmyl;
Cwy=p.Cwy;
yf=p.yf;
yt=p.yt;
xW=p.xW;
xf=p.xf;
xac=p.xac;
zW=p.zW;
yw=p.yw;
yW=p.yW;
yWE=p.yWE;
yWEE=p.yWEE;
K_omegaL=p.K_omegaL;
K_omegaR=p.K_omegaR;
K_deltaL=p.K_deltaL;
K_deltaR=p.K_deltaR;
CL_A=p.CL_A;
CL_B=p.CL_B;
CL_C=p.CL_C;
CD_A=p.CD_A;
CD_B=p.CD_B;
CD_C=p.CD_C;
CLB_A=p.CLB_A;
CLB_B=p.CLB_B;
CDB_A=p.CDB_A;
CDB_B=p.CDB_B;
% The constants below are for the polynomial approximations.
% I am lookin into a way of auto-generating them in a struct or something.
a11=p.a11;
a12=p.a12;
a13=p.a13;
a21=p.a21;
a22=p.a22;
a23=p.a23;
a31=p.a31;
a32=p.a32;
a33=p.a33;
a41=p.a41;
a42=p.a42;
a43=p.a43;
b11=p.b11;
b12=p.b12;
b13=p.b13;
b14=p.b14;
b21=p.b21;
b22=p.b22;
b23=p.b23;
b24=p.b24;
b31=p.b31;
b32=p.b32;
b33=p.b33;
b34=p.b34;
c11=p.c11;
c12=p.c12;
c13=p.c13;
c14=p.c14;
c21=p.c21;
c22=p.c22;
c23=p.c23;
c24=p.c24;
c31=p.c31;
c32=p.c32;
c33=p.c33;
c34=p.c34;
c41=p.c41;
c42=p.c42;
c43=p.c43;
c44=p.c44;
% Assuming we made correct choices here it should suffice with this:
%u = [u_deltaA u_jointA u_deltaT]';


% Hey, anyone reading this? Code below is auto-generated because the
% F.L. was just too much of a headache to do
% manyally, so I wrote a script for it.
wn = p.wn;
u_ref =[ ...
];
 
u_deltaA = u_ref(1);
u_jointA = u_ref(2);
u_deltaT = u_ref(3);

u_deltaL = u_jointA - u_deltaA/2;
u_deltaR = u_jointA + u_deltaA/2;
u_omegaL = u_jointT + u_deltaT/2;
u_omegaR = u_jointT - u_deltaT/2;

gain = 1;
u_deltaL = gain*u_deltaL;
u_deltaR = gain*u_deltaR;

end

== matlab function TailSitter_waypoints/TailSitter/tailsittersimv2 ==
  data: omegaLdot output; omegaRdot output; deltaLdot output; deltaRdot output; qdot output; wdot output; vdot output; omegaL input; omegaR input; deltaL input; deltaR input; u_omegaL input; u_omegaR input; u_deltaL input; u_deltaR input; q input; w input; v input; p parameter; alpha output; Beta output; g_out output
function [ omegaLdot, omegaRdot, deltaLdot, deltaRdot, qdot,wdot,vdot, alpha, Beta, g_out] = ...
    tailsitter_v2(omegaL, omegaR, deltaL, deltaR, u_omegaL, u_omegaR, u_deltaL, ...
    u_deltaR, q,w,v, p)

% Set output port dim
omegaLdot = 0;
omegaRdot = 0;
deltaLdot = 0;
deltaRdot = 0;
alpha = 0;
Beta = 0;
qdot = zeros(4,1);
wdot = zeros(3,1);
vdot = zeros(3,1);
g_out = zeros(3,1);

% Map inputs
vx = v(1);
vy = v(2);
vz = v(3);

wx = w(1);
wy = w(2);
wz = w(3);

q0 = q(1);
q1 = q(2);
q2 = q(3);
q3 = q(4);

% function handles not supported, so adding here directly
c = @(y) 0.28 - (0.28-0.09).*abs(y)./(p.b/2); % This should be pretty accurate
% Lift curves
CL = @(alpha) p.CL_A*sin(p.CL_B.*alpha)+p.CL_C; % These are wrong, just placeholders
CD = @(alpha) p.CD_A-p.CD_A.*cos(p.CD_B.*alpha)+p.CD_C;

alpha = atan2(vz,vx);

%Thrust
TL = p.K_T .* omegaL.^2;
TR = p.K_T .* omegaR.^2;

% airflow in thrust wake
v_w_L = p.b_w .* omegaL; %[b_w .* omegaL; vy; vz];
v_w_R = p.b_w .* omegaR;
%alpha_wL = atan2(vz,v_w_L);
%alpha_wR = atan2(vz,v_w_R);

% Quaternion
qdot = 0.5.*[-q1 -q2 -q3; ...
            q0 -q3 q2; ...
            q3 q0 -q1; ...
            -q2 q1 q0]*w;

% inputs
deltaLdot = p.K_deltaL .* (-deltaL + u_deltaL);
deltaRdot = p.K_deltaR .* (-deltaR + u_deltaR);
omegaLdot = p.K_omegaL .* (-omegaL + u_omegaL);
omegaRdot = p.K_omegaR .* (-omegaR + u_omegaR);

% gravity
% To get vector g in bf from wf
% we need to rotate it by q_wf, or conj(q_bf)
qc = quatconj([q0 q1 q2 q3]); %
qc0 = qc(1);
qc1 = qc(2);
qc2 = qc(3);
qc3 = qc(4);
gravity = p.g .* [2.*(qc1.*qc3 + qc0.*qc2); ...
                2.*(qc2.*qc3 - qc0.*qc1); ...
                (qc0.^2 - qc1.^2 - qc2.^2 + qc3.^2);
                zeros(3+4+4,1)];
g_out = gravity(1:3,1);
% Inertial forces
inertialF = -[2*(vz.*wy - vy.*wz); ...
             2*(vx.*wz - vz.*wx); ...
             2*(vy.*wx - vx.*wy); ...
             (p.Iz - p.Iy).*wy.*wz./p.Ix; ...
             (p.Ix - p.Iz).*wx.*wz./p.Iy; ...
             (p.Iy - p.Ix).*wx.*wy./p.Iz; ...
             zeros(8,1)];
%Sideslip
Beta = atan2(vy,vx);

% Winglets
CLB = @(beta) p.CLB_A*sin(p.CLB_B.*beta); % These are wrong, just placeholders
CDB = @(beta) p.CDB_A-p.CDB_A.*cos(p.CDB_B.*beta);
L_W = -p.rho * sqrt(vx.^2+vy.^2) * p.SW * (CLB(Beta)*vx + CDB(Beta)*vy); % Lift in bodyframe, y
D_W = p.rho * sqrt(vx.^2+vy.^2) * p.SW * (-CLB(Beta)*vy + CDB(Beta)*vx); % Drag in bodyfram, x

% MAIN WING
% Lift inside wake
LLT = p.Sw_w * 0.5 * p.rho * abs(v_w_L) .* CL(0).*v_w_L ;
LRT = p.Sw_w * 0.5 * p.rho * abs(v_w_R) .* CL(0).*v_w_R ;
% Lift outside wake
LL = p.Sw * 0.5 * p.rho * sqrt(vx.^2 + vz.^2) .* ...
    (CL(alpha).*vx + CD(alpha).*vz);
LR = LL; % Yeah we -could- combine these, but too late!
% Drag inside wake
DLT = p.Sw_w * 0.5 * p.rho * abs(v_w_L) * CD(0) * v_w_L;
DRT = p.Sw_w * 0.5 * p.rho * abs(v_w_R) * CD(0) * v_w_R;
% Drag outside wake
DL = p.Sw * 0.5 * p.rho * sqrt(vx.^2  + vz.^2) .* ...
    (-CL(alpha).*vz + CD(alpha).*vx);
DR = DL; % Yeah, we -could- combine these as well...

% AILERONS
% Lift inside wake, signs bc rotation dir of aileron
FLT = -p.CLdelta * 0.5*p.rho*v_w_L.^2 * p.Saw * deltaL;
FRT = -p.CLdelta * 0.5*p.rho*v_w_R.^2 * p.Saw * deltaR;
% Lift outside wake
FL = -sign(vx).*p.CLdelta * 0.5*p.rho*(vx.^2 + vy.^2 + vz.^2) * p.Sa * deltaL;
FR = -sign(vx).*p.CLdelta * 0.5*p.rho*(vx.^2 + vy.^2 + vz.^2) * p.Sa * deltaR;
% Drag inside wake
DalphaLT =p.CDdelta * 0.5*p.rho*v_w_L.^2 * p.Saw * abs(deltaL);
DalphaRT = p.CDdelta * 0.5*p.rho*v_w_R.^2 * p.Saw * abs(deltaR);
% Drag outside wake, we add sign of vx because we might be reversing?
DalphaL = sign(vx).*p.CDdelta * 0.5*p.rho*(vx.^2 + vy.^2 + vz.^2) * p.Sa * abs(deltaL);
DalphaR = sign(vx).*p.CDdelta * 0.5*p.rho*(vx.^2 + vy.^2 + vz.^2) * p.Sa * abs(deltaR);

% f1
 % diff in ail deflection
  % inside wake
  % outside wake
 % resmom roll,
 % roll due to yaw rate
 % moment due to sideslip
alphal_rmr = @(y) atan2(vz+wx.*y, vx);
restmomroll = @(y) y .* c(y) .* sqrt(vx.^2 + (vz+wx.*y).^2) .* ...
    (CL(alphal_rmr(y)).*vx + CD(alphal_rmr(y)).*(vz+wx.*y));
alphal_rwz = @(y) atan2(vz, vx-wz.*y);
rollduetowz = @(y) y .* c(y) .* sqrt((vx-wz.*y).^2 + vz.^2) .* ...
    (CL(alphal_rwz(y)).*(vx-wz*y) + CD(alphal_rwz(y)).*vz);
f1 = p.yf.*(FLT+FL -FRT-FR) ...
    -0.5*p.rho.*quadgk(restmomroll,-p.yW,p.yW) ... % between wakes
     -0.5*p.rho.*quadgk(restmomroll,-p.yWEE,-p.yWE) ... % outside left wake
      -0.5*p.rho.*quadgk(restmomroll,p.yWE,p.yWEE) ... % outside right wake
    -0.5*p.rho.*quadgk(rollduetowz,-p.yW,p.yW) ... between wakes
     -0.5*p.rho.*quadgk(rollduetowz,-p.yWEE,-p.yWE) ... left side
      -0.5*p.rho.*quadgk(rollduetowz, p.yWE,p.yWEE) ... right side
    +p.zW*L_W;
% f2
 % joint ail deflection
  % inside wake
  % outside wake
 % pitch moment
 % restmom pitch rate, --- compensate for wake!
 % Pitch from winglets
f2 = p.xf.*(FLT+FL+FRT+FR) ...
    ... %+ 0.5*p.rho*p.Cmyl*(2*p.Sw.*(vx.^2+vy.^2+vz.^2)+p.Sw_w*(v_w_L.^2 + v_w_R.^2) ) ...
    -p.xac.*(LL+LR+LLT+LRT) ... % We do not assume Pith coeff static.
    -wy.*p.rho.*2.*p.Sw.*p.Cwy.*sqrt(vx.^2 + vz.^2) ...
    +p.zW*D_W;
% f3
 % diff in T
 % mom due to sideslip
 % restmom yaw rate, compensate for outside wake
restmomwz = @(y) y .* c(y) .* sqrt((vx-wz.*y).^2 + vz.^2) .* ...
    (-CL(alphal_rwz(y)).*vz + CD(alphal_rwz(y)).*(vx-wz.*y));
f3 = p.yt.*(TL-TR) ...
     -p.xW*L_W ...
     +0.5*quadgk(restmomwz,-p.yW,p.yW) ...
     +0.5*quadgk(restmomwz,-p.yWEE,-p.yWE) ...
     +0.5*quadgk(restmomwz, p.yWE,p.yWEE);
 
%velocities
vxdot = (TL +TR -DL -DR -DLT -DRT -D_W -DalphaL -DalphaR -DalphaLT -DalphaRT)./p.m;
vydot = L_W./p.m;
vzdot = (-LL -LR -LLT -LRT +FL +FR +FLT +FRT)./p.m;

% angular rates
wxdot = f1./p.Ix;
wydot = f2./p.Iy;
wzdot = f3./p.Iz;

%if any(abs(vxdot) > 100)
%    p.m
%end

statesdot = gravity + inertialF +  ...
    [vxdot;vydot;vzdot;wxdot;wydot;wzdot;qdot;...
    deltaLdot;deltaRdot;omegaLdot;omegaRdot];

vdot = statesdot(1:3);
wdot = statesdot(4:6);
qdot = statesdot(7:10);
deltaLdot = statesdot(11);
deltaRdot = statesdot(12);
omegaLdot = statesdot(13);
omegaRdot = statesdot(14);

== matlab function TailSitter_waypoints/TailSitter/myQuatNorm ==
  data: q input; n output
function n = fcn(q)

n = sqrt(q(1).^2 + q(2).^2 + q(3).^2 + q(4).^2);

== matlab function TailSitter_waypoints/MATLAB Function ==
  data: u input; y output
function y = norm(u)

y = sqrt(sum(u.^2));

== matlab function TailSitter_waypoints/TailSitter/MATLAB Function ==
  data: time input; w output
function w = rotsteps(time)

stept = 10;
wt = 10;
reverse = 0;
if time<stept
    w = [0.1,0,0];
elseif time<stept+wt
    if reverse
        w = [-0.1,0,0];
    else
        w = zeros(1,3);
    end
elseif time<2*stept+wt
    w = [0,0,0.1];
elseif time<2*stept+2*wt
    if reverse
        w = [0,0,-0.1];
    else
        w = zeros(1,3);
    end
else
    w = [0,0.1,0];
end

== matlab function TailSitter_waypoints/MATLAB Function2 ==
  data: q_wf input; q_ref output
function q_ref = refquat(q_wf)

% TODO: Figure out how to set a good reference quaternion.
q_ref = q_wf;

== matlab function TailSitter_waypoints/MATLAB Function1 ==
  data: v_ref input; q_ref output; u_jointT output
function [q_ref,u_jointT] = ref_quat(v_ref)


q_ref = [1,0,0,0]';
u_jointT = 300;

% We have output of 5dof.
% Input is 3dof.
% We can extend input dof by saying we want wings to be horizontal, now
% total in is 4dof.


%Construct quaterion from several different rotations?
